simulink model "system3"  (R2018b)
settings: Solver=VariableStepAuto  StartTime=0.0  StopTime=10.0  RelTol=1e-3
libraries: cstblocks x7, simulink x2
settings Model: Creator=Abraham Pérez  LastModifiedBy=Abraham Pérez

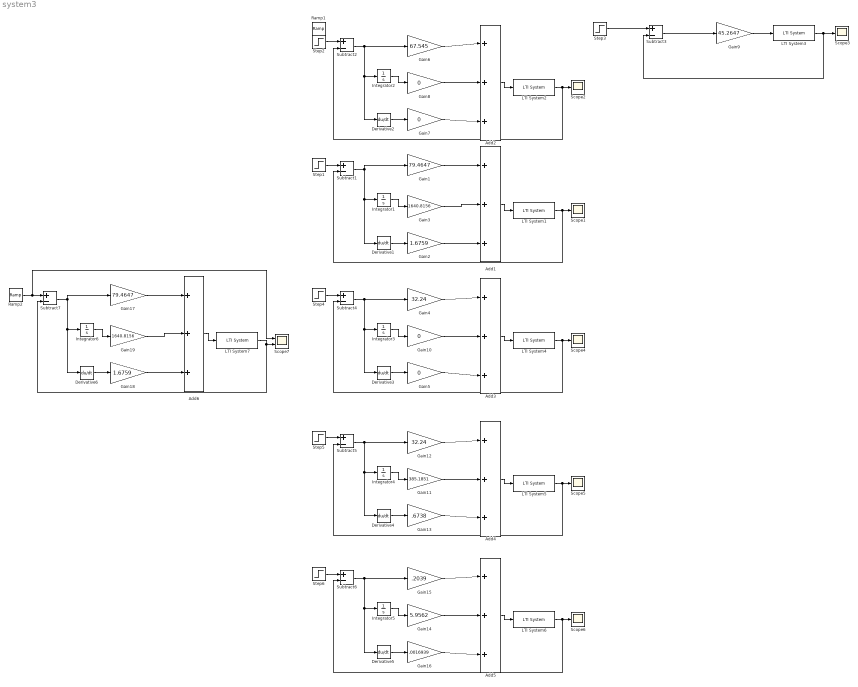
== system system3 ==
  Add{1..6} (6 alike) : Sum  Inputs=+++
  Derivative{1..6} (6 alike) : Derivative
  Gain1 : Gain  Gain=79.4647
  Gain{5,7..8,10} (4 alike) : Gain  Gain=0
  Gain11 : Gain  Gain=385.1851
  Gain12 : Gain  Gain=32.24
  Gain13 : Gain  Gain=.6738
  Gain14 : Gain  Gain=5.9562
  Gain15 : Gain  Gain=.2039
  Gain16 : Gain  Gain=.0016939
  Gain17 : Gain  Gain=79.4647
  Gain18 : Gain  Gain=1.6759
  Gain19 : Gain  Gain=1640.8156
  Gain2 : Gain  Gain=1.6759
  Gain3 : Gain  Gain=1640.8156
  Gain4 : Gain  Gain=32.24
  Gain6 : Gain  Gain=67.545
  Gain9 : Gain  Gain=45.2647
  Integrator{1..6} (6 alike) : Integrator
  LTI System{1..7} (7 alike) : cstblocks/LTI System  sys=G3  IC=[]
  Ramp1 : simulink/Sources/Ramp  slope=1  start=0  InitialOutput=17
  Ramp2 : simulink/Sources/Ramp  slope=1  start=0  InitialOutput=17
  Scope{1..6} (6 alike) : Scope
  Scope7 : Scope  NumInputPorts=2
  Step{1..2,4..6} (5 alike) : Step  Time=0  After=9  SampleTime=0
  Step3 : Step  Time=0  SampleTime=0
  Subtract{1..7} (7 alike) : Sum  Inputs=+-
  wires:
  Gain6/1 -> Add2/1
  Derivative2/1 -> Gain7/1
  LTI System2/1 -> Subtract2/2, Scope2/1
  Add2/1 -> LTI System2/1
  Integrator2/1 -> Gain8/1
  Step2/1 -> Subtract2/1
  Subtract2/1 -> Derivative2/1, Integrator2/1, Gain6/1
  Gain8/1 -> Add2/2
  Gain7/1 -> Add2/3
  LTI System3/1 -> Subtract3/2, Scope3/1
  Step3/1 -> Subtract3/1
  Gain9/1 -> LTI System3/1
  Subtract3/1 -> Gain9/1
  Derivative1/1 -> Gain2/1
  Gain1/1 -> Add1/1
  Gain3/1 -> Add1/2
  Integrator1/1 -> Gain3/1
  Gain2/1 -> Add1/3
  Subtract1/1 -> Derivative1/1, Integrator1/1, Gain1/1
  Step1/1 -> Subtract1/1
  LTI System1/1 -> Subtract1/2, Scope1/1
  Add1/1 -> LTI System1/1
  Derivative3/1 -> Gain5/1
  Gain4/1 -> Add3/1
  Gain10/1 -> Add3/2
  Integrator3/1 -> Gain10/1
  Gain5/1 -> Add3/3
  Subtract4/1 -> Derivative3/1, Integrator3/1, Gain4/1
  Step4/1 -> Subtract4/1
  LTI System4/1 -> Subtract4/2, Scope4/1
  Add3/1 -> LTI System4/1
  Add4/1 -> LTI System5/1
  Step5/1 -> Subtract5/1
  LTI System5/1 -> Subtract5/2, Scope5/1
  Subtract5/1 -> Derivative4/1, Integrator4/1, Gain12/1
  Gain13/1 -> Add4/3
  Gain11/1 -> Add4/2
  Integrator4/1 -> Gain11/1
  Derivative4/1 -> Gain13/1
  Gain12/1 -> Add4/1
  Gain14/1 -> Add5/2
  Derivative5/1 -> Gain16/1
  Gain15/1 -> Add5/1
  Add5/1 -> LTI System6/1
  Gain16/1 -> Add5/3
  LTI System6/1 -> Subtract6/2, Scope6/1
  Subtract6/1 -> Derivative5/1, Integrator5/1, Gain15/1
  Step6/1 -> Subtract6/1
  Integrator5/1 -> Gain14/1
  Gain19/1 -> Add6/2
  Gain18/1 -> Add6/3
  LTI System7/1 -> Subtract7/2, Scope7/2
  Integrator6/1 -> Gain19/1
  Subtract7/1 -> Derivative6/1, Integrator6/1, Gain17/1
  Gain17/1 -> Add6/1
  Derivative6/1 -> Gain18/1
  Add6/1 -> LTI System7/1
  Ramp2/1 -> Scope7/1, Subtract7/1
